simulink model "moment"  (R2021b)
settings: Solver=VariableStepAuto  StartTime=0.0  StopTime=5  RelTol=1e-3
libraries: shared6dof x1, aerolibanim x1, matrix_library x1
settings Model: Creator=josepfamador  LastModifiedBy=josepfamador

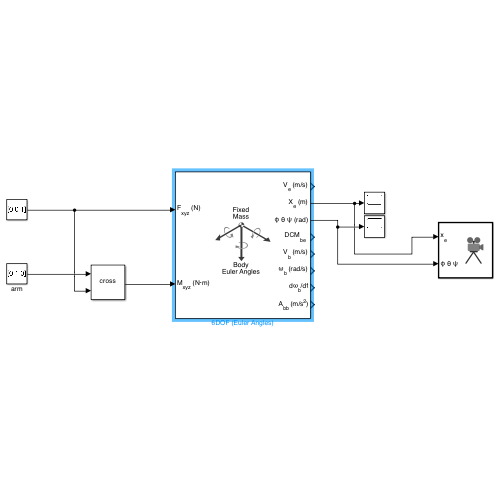
[thumbnail: Simulink's stored preview of the top-level diagram]
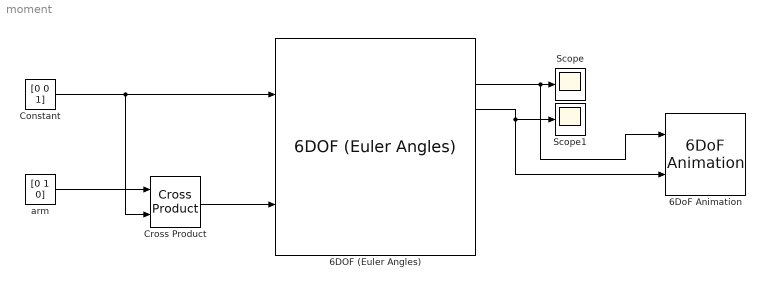
== system moment ==
  6DOF (Euler Angles) : shared6dof/6DOF (Euler Angles)  units=Metric (MKS)  mtype=Fixed  rep=Euler Angles  xme_0=[0 0 0]  Vm_0=[0 0 0]  eul_0=[0 0 0]  pm_0=[0 0 0]  mass_0=1.0  mass_e=0.5  mass_f=2.0  inertia=eye(3)  inertia_e=eye(3)  inertia_f=2*eye(3)  k_quat=1.0  vre_flag=on  abi_flag=off  aMode=0  xme_statename=''  Vm_statename=''  eul_statename=''  quat_statename=''  pm_statename=''  mass_statename=''
      settings: SourceProductBaseCode=AE,PW,DR,MT,UV,VE
  6DoF Animation : aerolibanim/6DoF Animation  u1=[0 4000 -2000 2000 -5000 -3000]  u2=0.1  u3=1.0  u4=[4000 0 -5000]  u5=Fixed position  u6=[2000 500 -3150]  u7=10  u8=on
  Constant : Constant  Value=[0 0 1]
  Cross Product : matrix_library/Cross Product
      settings: SourceProductBaseCode=SL
  Scope : Scope
  Scope1 : Scope
  arm : Constant  Value=[0 1 0]
  wires:
  6DOF (Euler Angles)/2 -> 6DoF Animation/1, Scope/1
  6DOF (Euler Angles)/3 -> 6DoF Animation/2, Scope1/1
  Constant/1 -> Cross Product/2, 6DOF (Euler Angles)/1
  arm/1 -> Cross Product/1
  Cross Product/1 -> 6DOF (Euler Angles)/2
